simulink library "phase_shift_filter_ccaller"  (R2025b)
settings: Solver=VariableStepAuto  StartTime=0.0  StopTime=10.0  RelTol=1e-3
undefined symbols (not defined in the file): frequency_set, ts_inv
settings Model: Creator=dbagn  LastModifiedBy=dbagn
settings SFSimCC: SimCustomHeaderCode=|
  | #include "phase_shift_flt_simulink.h"
  | #include "phase_shift_flt.h"
settings SFSimCC: SimUserSources=|
  | "phase_shift_flt_simulink.c"
  | "phase_shift_flt.c"
settings SFSimCC: SimUserIncludeDirs=|
  | include
  | src

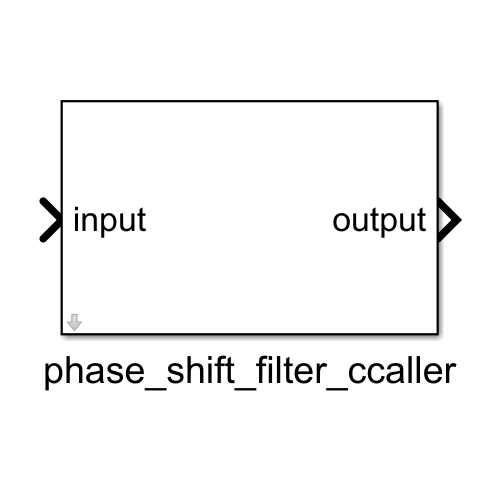
[thumbnail: Simulink's stored preview of the top-level diagram]
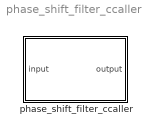
== system phase_shift_filter_ccaller ==
  phase_shift_filter_ccaller : Subsystem  mask{freq_m=frequency_set, ts_m=ts_inv, scaling_m=1 %phase_shift_filter_gain, reset_time_release=0.025, instance=0, tc_m=-1}
      mask prompts: freq_m "Frequency at 90 degPhase Shift [Hz]"; ts_m "Sampling Time [s]"; scaling_m "Scaling Output (correction)"; reset_time_release "Reset Time Release [s]"; tc_m "Sample Time [-1] (-1 for inherited)"

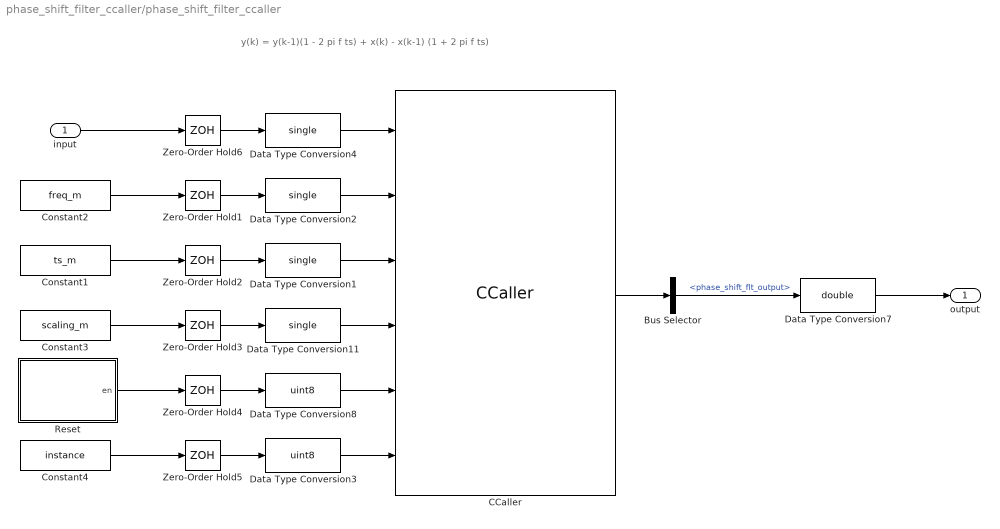
== system phase_shift_filter_ccaller/phase_shift_filter_ccaller ==
  note: y(k) = y(k-1)(1 - 2 pi f ts) + x(k) - x(k-1) (1 + 2 pi f ts)
  input : Inport
  Bus Selector : BusSelector  OutputSignals=phase_shift_flt_output
  CCaller : CCaller  FunctionName=phase_shift_flt_process_simulink  PortSpecificationStruct="%)30     .    , P   8    (     @         %    \"     <    !     0         %  0 \"0    $    _    07)G3F%M90  4&]R=$YA;64 4V-O<&4     26YD97@     5'EP90      4VEZ90      27-';&]B86P   X    P    !@    @    $          4    (     0    ,    !         !   P!O=70 #@   #     &    \"     0         !0    @    !     P    $         $  # &]U=  .    .     8    (    !          %    \"     $    &     0         0   ...(+3823 chars)"  SampleTime=tc_m
  Constant1 : Constant  Value=ts_m
  Constant2 : Constant  Value=freq_m
  Constant3 : Constant  Value=scaling_m
  Constant4 : Constant  Value=instance
  Data Type Conversion{1..2,4,11} (4 alike) : DataTypeConversion  OutDataTypeStr=single  SaturateOnIntegerOverflow=off  RndMeth=Floor
  Data Type Conversion3 : DataTypeConversion  OutDataTypeStr=uint8  SaturateOnIntegerOverflow=off  RndMeth=Floor
  Data Type Conversion7 : DataTypeConversion  OutDataTypeStr=double  SaturateOnIntegerOverflow=off  RndMeth=Floor
  Data Type Conversion8 : DataTypeConversion  OutDataTypeStr=uint8  SaturateOnIntegerOverflow=off  RndMeth=Floor
  Reset : Subsystem
  Zero-Order Hold{1..6} (6 alike) : ZeroOrderHold  SampleTime=tc_m
  output : Outport
  wires:
  Zero-Order Hold6/1 -> Data Type Conversion4/1
  Data Type Conversion7/1 -> output/1
  Data Type Conversion4/1 -> CCaller/1
  Bus Selector/1 -> Data Type Conversion7/1  "<phase_shift_flt_output>"
  CCaller/1 -> Bus Selector/1
  Constant4/1 -> Zero-Order Hold5/1
  Data Type Conversion3/1 -> CCaller/6
  Zero-Order Hold5/1 -> Data Type Conversion3/1
  Data Type Conversion2/1 -> CCaller/2
  Constant2/1 -> Zero-Order Hold1/1
  Zero-Order Hold1/1 -> Data Type Conversion2/1
  Data Type Conversion1/1 -> CCaller/3
  Zero-Order Hold2/1 -> Data Type Conversion1/1
  Constant1/1 -> Zero-Order Hold2/1
  Data Type Conversion8/1 -> CCaller/5
  Reset/1(en) -> Zero-Order Hold4/1
  Zero-Order Hold4/1 -> Data Type Conversion8/1
  Constant3/1 -> Zero-Order Hold3/1
  Zero-Order Hold3/1 -> Data Type Conversion11/1
  Data Type Conversion11/1 -> CCaller/4
  input/1 -> Zero-Order Hold6/1

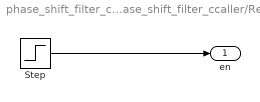
== system phase_shift_filter_ccaller/phase_shift_filter_ccaller/Reset ==
  Step : Step  Time=reset_time_release  Before=1  After=0  SampleTime=tc_m
  en : Outport
  wires:
  Step/1 -> en/1
